simulink library "lib_affectiveChar_scenario"  (R2014a)
settings: Solver=ode45  StartTime=0.0  StopTime=10.0  RelTol=1e-3
values from neighbouring files (symbols this model uses):
  temp = sprintf('<face type=\"FACS\" side=\"BOTH\" au=\"    [cmdBML_AU.m]    (also in cmdBML_AU_VA.m; cmdBML_AUmerg.m; cmdBML_AUs.m)
undefined symbols (not defined in the file or in its folder): avert, bHand, boredom, BOREDOM_THRESHOLD, diff, GAZE_GUI, GAZE_SHOFTEYE, GAZE_USER_HAND, gazing, isPosing, p, r, randAvertGazeChance, randPoseChance, s, uHand
(part 1 of 2)
settings Model: Creator=Maryam  LastModifiedBy=root180

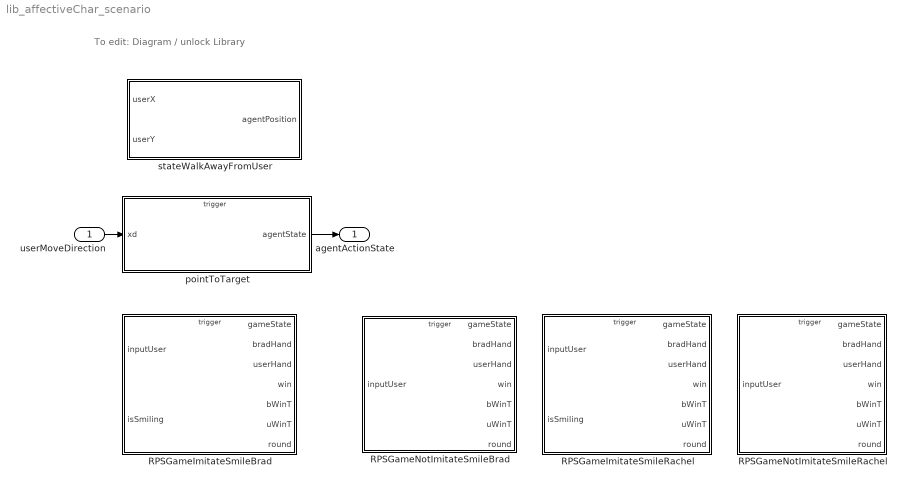
== system lib_affectiveChar_scenario ==
  note: To edit: Diagram / unlock Library
  userMoveDirection : Inport
  RPSGameImitateSmileBrad : Stateflow chart  TreatAsAtomicUnit=on
  RPSGameImitateSmileRachel : Stateflow chart  TreatAsAtomicUnit=on  DSMNames=BOREDOM_THRESHOLD,GAZE_GUI,GAZE_SHOFTEYE,GAZE_USER_HAND,avert,bHand,boredom,diff,gazing,isPosing,p,r,randAvertGazeChance,randPoseChance,s,temp,uHand  DSMValues=BOREDOM_THRESHOLD,GAZE_GUI,GAZE_SHOFTEYE,GAZE_USER_HAND,avert,bHand,boredom,diff,gazing,isPosing,p,r,randAvertGazeChance,randPoseChance,s,temp,uHand
  RPSGameNotImitateSmileBrad : Stateflow chart  TreatAsAtomicUnit=on
  RPSGameNotImitateSmileRachel : Stateflow chart  TreatAsAtomicUnit=on
  pointToTarget : Stateflow chart  TreatAsAtomicUnit=on
  stateWalkAwayFromUser : Stateflow chart  TreatAsAtomicUnit=on
  agentActionState : Outport
  wires:
  userMoveDirection/1 -> pointToTarget/1(xd)
  pointToTarget/1(agentState) -> agentActionState/1

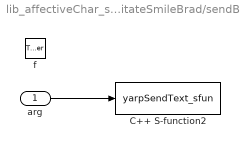
== system lib_affectiveChar_scenario/RPSGameImitateSmileBrad/sendBML ==
  arg : Inport  OutDataTypeStr=double  PortDimensions=[256 1]
  f : TriggerPort  TriggerType=function-call
      settings: CopyFcn=Stateflow.SLINSF.SimulinkMan.removeBlockPreDeleteFcn  PreDeleteFcn=Stateflow.SLINSF.SimulinkMan.unsafePredeleteFcn
  C++ S-function2 : S-Function  FunctionName=yarpSendText_sfun  Parameters='/sim/out/bml0', '/SB/in/bml'  EnableBusSupport=off
  wires:
  arg/1 -> C++ S-function2/1

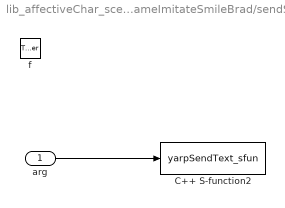
== system lib_affectiveChar_scenario/RPSGameImitateSmileBrad/sendSBM ==
  arg : Inport  OutDataTypeStr=double  PortDimensions=[256 1]
  f : TriggerPort  TriggerType=function-call
      settings: CopyFcn=Stateflow.SLINSF.SimulinkMan.removeBlockPreDeleteFcn  PreDeleteFcn=Stateflow.SLINSF.SimulinkMan.unsafePredeleteFcn
  C++ S-function2 : S-Function  FunctionName=yarpSendText_sfun  Parameters='/sim/out/smb0', '/SB/in/sbm'  EnableBusSupport=off
  wires:
  arg/1 -> C++ S-function2/1

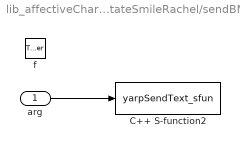
== system lib_affectiveChar_scenario/RPSGameImitateSmileRachel/sendBML ==
  arg : Inport  OutDataTypeStr=double  PortDimensions=[256 1]
  f : TriggerPort  TriggerType=function-call
      settings: CopyFcn=Stateflow.SLINSF.SimulinkMan.removeBlockPreDeleteFcn  PreDeleteFcn=Stateflow.SLINSF.SimulinkMan.unsafePredeleteFcn
  C++ S-function2 : S-Function  FunctionName=yarpSendText_sfun  Parameters='/sim/out/bml0', '/SB/in/bml'  EnableBusSupport=off
  wires:
  arg/1 -> C++ S-function2/1

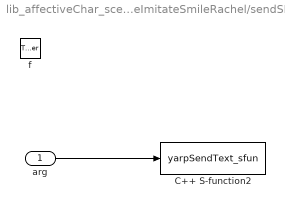
== system lib_affectiveChar_scenario/RPSGameImitateSmileRachel/sendSBM ==
  arg : Inport  OutDataTypeStr=double  PortDimensions=[256 1]
  f : TriggerPort  TriggerType=function-call
      settings: CopyFcn=Stateflow.SLINSF.SimulinkMan.removeBlockPreDeleteFcn  PreDeleteFcn=Stateflow.SLINSF.SimulinkMan.unsafePredeleteFcn
  C++ S-function2 : S-Function  FunctionName=yarpSendText_sfun  Parameters='/sim/out/smb0', '/SB/in/sbm'  EnableBusSupport=off
  wires:
  arg/1 -> C++ S-function2/1

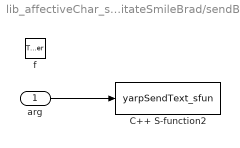
== system lib_affectiveChar_scenario/RPSGameNotImitateSmileBrad/sendBML ==
  arg : Inport  OutDataTypeStr=double  PortDimensions=[256 1]
  f : TriggerPort  TriggerType=function-call
      settings: CopyFcn=Stateflow.SLINSF.SimulinkMan.removeBlockPreDeleteFcn  PreDeleteFcn=Stateflow.SLINSF.SimulinkMan.unsafePredeleteFcn
  C++ S-function2 : S-Function  FunctionName=yarpSendText_sfun  Parameters='/sim/out/bml0', '/SB/in/bml'  EnableBusSupport=off
  wires:
  arg/1 -> C++ S-function2/1

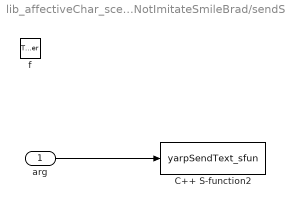
== system lib_affectiveChar_scenario/RPSGameNotImitateSmileBrad/sendSBM ==
  arg : Inport  OutDataTypeStr=double  PortDimensions=[256 1]
  f : TriggerPort  TriggerType=function-call
      settings: CopyFcn=Stateflow.SLINSF.SimulinkMan.removeBlockPreDeleteFcn  PreDeleteFcn=Stateflow.SLINSF.SimulinkMan.unsafePredeleteFcn
  C++ S-function2 : S-Function  FunctionName=yarpSendText_sfun  Parameters='/sim/out/smb0', '/SB/in/sbm'  EnableBusSupport=off
  wires:
  arg/1 -> C++ S-function2/1

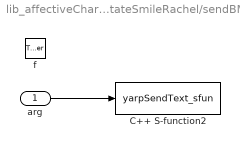
== system lib_affectiveChar_scenario/RPSGameNotImitateSmileRachel/sendBML ==
  arg : Inport  OutDataTypeStr=double  PortDimensions=[256 1]
  f : TriggerPort  TriggerType=function-call
      settings: CopyFcn=Stateflow.SLINSF.SimulinkMan.removeBlockPreDeleteFcn  PreDeleteFcn=Stateflow.SLINSF.SimulinkMan.unsafePredeleteFcn
  C++ S-function2 : S-Function  FunctionName=yarpSendText_sfun  Parameters='/sim/out/bml0', '/SB/in/bml'  EnableBusSupport=off
  wires:
  arg/1 -> C++ S-function2/1

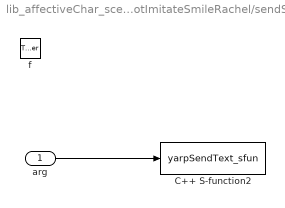
== system lib_affectiveChar_scenario/RPSGameNotImitateSmileRachel/sendSBM ==
  arg : Inport  OutDataTypeStr=double  PortDimensions=[256 1]
  f : TriggerPort  TriggerType=function-call
      settings: CopyFcn=Stateflow.SLINSF.SimulinkMan.removeBlockPreDeleteFcn  PreDeleteFcn=Stateflow.SLINSF.SimulinkMan.unsafePredeleteFcn
  C++ S-function2 : S-Function  FunctionName=yarpSendText_sfun  Parameters='/sim/out/smb0', '/SB/in/sbm'  EnableBusSupport=off
  wires:
  arg/1 -> C++ S-function2/1

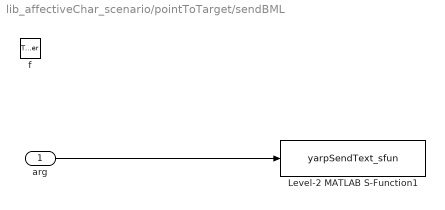
== system lib_affectiveChar_scenario/pointToTarget/sendBML ==
  arg : Inport  OutDataTypeStr=double  PortDimensions=[256 1]
  f : TriggerPort  TriggerType=function-call
      settings: CopyFcn=Stateflow.SLINSF.SimulinkMan.removeBlockPreDeleteFcn  PreDeleteFcn=Stateflow.SLINSF.SimulinkMan.unsafePredeleteFcn
  Level-2 MATLAB S-Function1 : M-S-Function  FunctionName=yarpSendText_sfun  Parameters='/sim/out/bml', '/SB/in/bml'
  wires:
  arg/1 -> Level-2 MATLAB S-Function1/1

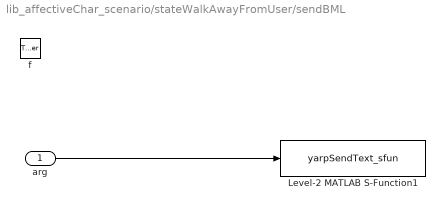
== system lib_affectiveChar_scenario/stateWalkAwayFromUser/sendBML ==
  arg : Inport  OutDataTypeStr=double  PortDimensions=[256 1]
  f : TriggerPort  TriggerType=function-call
      settings: CopyFcn=Stateflow.SLINSF.SimulinkMan.removeBlockPreDeleteFcn  PreDeleteFcn=Stateflow.SLINSF.SimulinkMan.unsafePredeleteFcn
  Level-2 MATLAB S-Function1 : M-S-Function  FunctionName=yarpSendText_sfun  Parameters='/sim/out/bml4', '/SB/in/bml'
  wires:
  arg/1 -> Level-2 MATLAB S-Function1/1

== stateflow chart lib_affectiveChar_scenario/stateWalkAwayFromUser ==
  state stateWalkAway
    entry:
    [arrBML,agentPosition ] = cmdBML_walkOppositeUser(userX, userY);
    sendBML(arrBML);
  state sendBML(arg) [function]
  data: arg function_input double size=[256 1]; userX input =5; userY input =5; agentPosition output double size=1; arrBML data_store_memory size=256

== stateflow chart lib_affectiveChar_scenario/RPSGameImitateSmileBrad ==
  state stateStart
    entry: round=0;avert=0;
    uHand=1; randSmile=0; userHand=3;bradHand=3; win=0;
    BOREDOM_THRESHOLD=10;
    gameState=0;randPoseChance=0;randAvertGazeChance=0;
    uWinT=0; bWinT=0; isPosing=0;
    boredom=0;
    sendBML(  initialPoseTable(1) );
  state sendSBM(arg) [function]
  state stateReady
    entry: round=round+1;
    bradHand=3;
    userHand=3;
    gameState= 0;
    win=0;isPosing=1;
  state sendBML(arg) [function]
  note: num of bmlID=2
  state gameOver
    entry: gameState=3;
    boredom=boredom-2;
  note: num of bmlID=2
  state statePoseReady
    entry:
    sendBML(  initialPoseTable(2) );
    sendSBM(handPoseSBTable(2));
    isPosing=1;
  note: num of bmlID=2
  state stateHeadNeutral2
    entry:
    sendBML( initialPoseTable(2 ) );
  note: num of sbmID=4
  note: num of bmlID=18
  state stateGo
    entry: isPosing=1;
    gameState= 1;
  state stateWinSmile
    entry:
    sendBML(successTable(1));
  note: num of bmlID=3
  state stateNeckBack
    entry: sendBML( successTable(2));
  state stateRandomHand
    entry: isPosing=1;
    bHand=randi([0,2]);
  state stateBrowUp
    entry:  sendBML( successTable(3));
  state statePoseFingersCLose
    entry:isPosing=1;
    sendSBM(handPoseSBTable(1));
  state stateNotWinBored
    entry:
    sendBML( idlePoseBradTable(randi([1,18])) );
  state statePosePaper
    entry: isPosing=1;p=randi([1,2]);
    sendBML(  paperPoseBradTable(p) );
  state statePoseRock
    entry: isPosing=1;r=randi([1,2]);
    sendBML(  rockPoseTable(r) );
  state statePoseScissors
    entry: isPosing=1; s=randi([1,2]);
    sendBML(  scissorsPoseBradTable(s) );
  state stateReadUserHand
    entry:isPosing=1;
    uHand=inputUser;
  state stateShowHands
    entry: isPosing=1;
    gameState=2;
    bradHand=bHand;
    userHand=uHand;
  state statePoseReturnFinger
    entry:isPosing=1;
    sendSBM(handPoseSBTable(2));
  state stateCompare
    entry:isPosing=1;
    temp=uHand-bHand;
    diff=temp- 3.*floor(temp/3);
  state stateUserWin
    entry:isPosing=0;
    win=1;
    uWinT=uWinT+1;
  state stateBradWin
    entry:isPosing=0;
    win=2;
    bWinT=bWinT+1;
  state stateNoWin
    entry:
    win=0;
    isPosing=0;
  state stateShowResult
    entry: isPosing=0;
  (default) -> stateStart
  stateStart -> stateReady : after(2,secs)
  stateReady -> stateReady [order 2] : [uHand==3]
  stateReady -> statePoseReady [order 1] : after(1,secs)[boredom<BOREDOM_THRESHOLD-4]{boredom=boredom+1;}
  (junction 2) -> stateReady [order 2] : after(3,secs)
  stateReady -> statePoseReady [order 3] : after(1,secs)
  (junction 2) -> gameOver [order 1] : after(3,secs)[round==10]
  stateShowResult -> (junction 2)
  gameOver -> stateHeadNeutral2
  stateHeadNeutral2 -> (junction 3) : after(1,secs)
  statePoseReady -> stateGo : after(3,secs)[uHand~=3]
  (junction 3) -> stateWinSmile [order 1] : [uWinT<bWinT]
  (junction 3) -> stateNotWinBored [order 2]
  stateWinSmile -> stateNeckBack : after(1,secs)
  stateGo -> stateRandomHand : after(1,secs)
  stateNeckBack -> stateBrowUp : after(1,secs)
  stateRandomHand -> (junction 5)
  (junction 5) -> statePoseFingersCLose [order 3] : [bHand==0]
  (junction 5) -> statePoseRock [order 2] : [bHand==2]
  (junction 5) -> statePosePaper [order 1] : [bHand==1]
  statePoseFingersCLose -> statePoseScissors
  statePoseRock -> stateReadUserHand : after(1,secs)[uHand~=3]
  statePosePaper -> stateReadUserHand : after(1,secs)[uHand~=3]
  statePoseScissors -> stateReadUserHand : after(1,secs)[uHand~=3]
  stateReadUserHand -> stateReadUserHand [order 1] : [uHand==3]
  stateReadUserHand -> statePoseReturnFinger [order 2] : [bHand==0]
  stateReadUserHand -> stateShowHands [order 3]
  statePoseReturnFinger -> stateShowHands
  stateShowHands -> stateCompare
  stateCompare -> stateUserWin [order 2] : [diff==2]
  stateCompare -> stateBradWin [order 1] : [diff==1]
  stateCompare -> stateNoWin [order 3] : [diff~=1 && diff~=2]
  stateBradWin -> stateShowResult
  stateNoWin -> stateShowResult : after(5,secs)
  stateUserWin -> stateShowResult : after(5,secs)
  data: arg function_input double size=[256 1]; arg function_input double size=[256 1]; bmlID function_input double; poseBML function_output double size=[256,1]; bmlID function_input double; poseBML function_output double size=[256,1]; bmlID function_input double; poseBML function_output double size=[256,1]; sbmID function_input double; poseSBM function_output double size=[256,1]; bmlID function_input double; poseBML function_output double size=[256,1]; bmlID function_input double; poseBML function_output double size=[256,1]; bmlID function_input double; poseBML function_output double size=[256,1]; gameState output double size=1 =0; inputUser input double size=1; bradHand output double size=1; userHand output double size=1 =3; win output double size=1; temp data_store_memory size=2; diff data_store_memory size=2; uHand data_store_memory size=2; bHand data_store_memory size=2; bWinT output double size=1; uWinT output double size=1; smileN data_store_memory size=2; randSmile data_store_memory size=2; boredom data_store_memory size=2; BOREDOM_THRESHOLD data_store_memory size=2; randAvertGazeChance data_store_memory size=2; randPoseChance data_store_memory size=2; isPosing data_store_memory size=2; r data_store_memory size=2; p data_store_memory size=2; s data_store_memory size=2; round output double size=1 =0; isSmiling input double size=1; avert data_store_memory
  events: secs input RISING_EDGE_EVENT
  function poseBML = rockPoseTable(bmlID):
    | function poseBML = rockPoseTable(bmlID)
    | 
    | aVarTruthTableCondition_1 = false;
    | aVarTruthTableCondition_2 = false;
    | 
    | 
    | % rock
    | 
    | aVarTruthTableCondition_1 = logical(bmlID==1);
    | 
    | % rock
    | 
    | aVarTruthTableCondition_2 = logical(bmlID==2);
    | 
    | if (aVarTruthTableCondition_1)
    |     aFcnTruthTableAction_1();
    | elseif (aVarTruthTableCondition_2)
    |     aFcnTruthTableAction_2();
    | else % Default
    |     aFcnTruthTableAction_1();
    | end
    | 
    | function aFcnTruthTableAction_1()
    | 
    | % rock
    | 
    | poseBML=encStr2Arr('<?xml version="1.0" ?><act><bml><animation name="ChrBrad@Idle01_BeatFistMidLf02"/></bml></act>');
    | 
    | function aFcnTruthTableAction_2()
    | 
    | % rock2
    | 
    | poseBML=encStr2Arr('<?xml version="1.0" ?><act><bml><animation name="ChrBrad@Idle01_BeatFistMidLf01"/></bml></act>');
  function poseBML = paperPoseBradTable(bmlID):
    | function poseBML = paperPoseBradTable(bmlID)
    | 
    | aVarTruthTableCondition_1 = false;
    | aVarTruthTableCondition_2 = false;
    | 
    | 
    | % paper
    | 
    | aVarTruthTableCondition_1 = logical(bmlID==1);
    | 
    | % paper2
    | 
    | aVarTruthTableCondition_2 = logical(bmlID==2);
    | 
    | if (aVarTruthTableCondition_1)
    |     aFcnTruthTableAction_1();
    | elseif (aVarTruthTableCondition_2)
    |     aFcnTruthTableAction_2();
    | else % Default
    |     aFcnTruthTableAction_2();
    | end
    | 
    | function aFcnTruthTableAction_1()
    | 
    | % paper
    | 
    | poseBML=encStr2Arr('<?xml version="1.0" ?><act><bml><animation name="ChrBrad@Idle01_OfferLf01"/></bml></act>');
    | 
    | function aFcnTruthTableAction_2()
    | 
    | % paper2
    | 
    | poseBML=encStr2Arr('<?xml version="1.0" ?><act><bml><animation name="ChrBrad@Idle01_YouLf01"/></bml></act>');
  function poseBML = scissorsPoseBradTable(bmlID):
    | function poseBML = scissorsPoseBradTable(bmlID)
    | 
    | aVarTruthTableCondition_1 = false;
    | aVarTruthTableCondition_2 = false;
    | 
    | 
    | % scissors
    | 
    | aVarTruthTableCondition_1 = logical(bmlID==1);
    | 
    | % scissors2
    | 
    | aVarTruthTableCondition_2 = logical(bmlID==2);
    | 
    | if (aVarTruthTableCondition_1)
    |     aFcnTruthTableAction_1();
    | elseif (aVarTruthTableCondition_2)
    |     aFcnTruthTableAction_2();
    | else % Default
    |     aFcnTruthTableAction_1();
    | end
    | 
    | function aFcnTruthTableAction_1()
    | 
    | % scissors
    | 
    | poseBML=encStr2Arr('<?xml version="1.0" ?><act><bml><animation name="ChrBrad@Idle01_YouLf01"/></bml></act>');
    | 
    | function aFcnTruthTableAction_2()
    | 
    | % scissors2
    | 
    | poseBML=encStr2Arr('<?xml version="1.0" ?><act><bml><animation name="ChrBrad@Idle01_OfferLf01"/></bml></act>');
  function poseSBM = handPoseSBTable(sbmID):
    | function poseSBM = handPoseSBTable(sbmID)
    | 
    | aVarTruthTableCondition_1 = false;
    | aVarTruthTableCondition_2 = false;
    | aVarTruthTableCondition_3 = false;
    | aVarTruthTableCondition_4 = false;
    | 
    | 
    | % fingersClose
    | 
    | aVarTruthTableCondition_1 = logical(sbmID==1);
    | 
    | % fingersNeutral
    | 
    | aVarTruthTableCondition_2 = logical(sbmID==2);
    | 
    | % lshoulkderForward
    | 
    | aVarTruthTableCondition_3 = logical(sbmID==3);
    | 
    | % lshoulkderNeutral
    | 
    | aVarTruthTableCondition_4 = logical(sbmID==4);
    | 
    | if (aVarTruthTableCondition_1)
    |     aFcnTruthTableAction_1();
    | elseif (aVarTruthTableCondition_2)
    |     aFcnTruthTableAction_2();
    | elseif (aVarTruthTableCondition_3)
    |     aFcnTruthTableAction_3();
    | elseif (aVarTruthTableCondition_4)
    |     aFcnTruthTableAction_4();
    | else % Default
    |     aFcnTruthTableAction_1();
    | end
    | 
    | function aFcnTruthTableAction_1()
    | 
    | % fingersClose
    | 
    | poseSBM=encStr2Arr('brad.getSkeleton().getJointByName("l_pinky1").setPostrotation(SrQuat(1,0,0,0.5)); brad.getSkeleton().getJointByName("l_ring1").setPostrotation(SrQuat(1,0,0,0.5))');
    | 
    | function aFcnTruthTableAction_2()
    | 
    | % fingersNeutral
    | 
    | poseSBM=encStr2Arr('brad.getSkeleton().getJointByName("l_pinky1").setPostrotation(SrQuat(1,0,0,0)); brad.getSkeleton().getJointByName("l_ring1").setPostrotation(SrQuat(1,0,0,0))');
    | 
    | function aFcnTruthTableAction_3()
    | 
    | % lshoulkderForward
    | 
    | poseSBM=encStr2Arr('brad.getSkeleton().getJointByName("l_sternoclavicular").setPostrotation(SrQuat(1,0,0,0.05))');
    | 
    | function aFcnTruthTableAction_4()
    | 
    | % lshoulkderNeutral
    | 
    | poseSBM=encStr2Arr('brad.getSkeleton().getJointByName("l_sternoclavicular").setPostrotation(SrQuat(1,0,0,0))');
  function poseBML=idlePoseBradTable(bmlID):
    | function poseBML=idlePoseBradTable(bmlID)
    | 
    | aVarTruthTableCondition_1 = false;
    | aVarTruthTableCondition_2 = false;
    | aVarTruthTableCondition_3 = false;
    | aVarTruthTableCondition_4 = false;
    | aVarTruthTableCondition_5 = false;
    | aVarTruthTableCondition_6 = false;
    | aVarTruthTableCondition_7 = false;
    | aVarTruthTableCondition_8 = false;
    | aVarTruthTableCondition_9 = false;
    | aVarTruthTableCondition_10 = false;
    | aVarTruthTableCondition_11 = false;
    | aVarTruthTableCondition_12 = false;
    | aVarTruthTableCondition_13 = false;
    | aVarTruthTableCondition_14 = false;
    | aVarTruthTableCondition_15 = false;
    | aVarTruthTableCondition_16 = false;
    | aVarTruthTableCondition_17 = false;
    | aVarTruthTableCondition_18 = false;
    | 
    | 
    | 
    | aVarTruthTableCondition_1 = logical(bmlID==1);
    | 
    | 
    | aVarTruthTableCondition_2 = logical(bmlID==2);
    | 
    | 
    | aVarTruthTableCondition_3 = logical(bmlID==3);
    | 
    | 
    | aVarTruthTableCondition_4 = logical(bmlID==4);
    | 
    | 
    | aVarTruthTableCondition_5 = logical(bmlID==5);
    | 
    | 
    | aVarTruthTableCondition_6 = logical(bmlID==6);
    | 
    | 
    | aVarTruthTableCondition_7 = logical(bmlID==7);
    | 
    | 
    | aVarTruthTableCondition_8 = logical(bmlID==8);
    | 
    | 
    | aVarTruthTableCondition_9 = logical(bmlID==9);
    | 
    | 
    | aVarTruthTableCondition_10 = logical(bmlID==10);
    | 
    | 
    | aVarTruthTableCondition_11 = logical(bmlID==11);
    | 
    | 
    | aVarTruthTableCondition_12 = logical(bmlID==12);
    | 
    | 
    | aVarTruthTableCondition_13 = logical(bmlID==13);
    | 
    | 
    | aVarTruthTableCondition_14 = logical(bmlID==14);
    | 
    | 
    | aVarTruthTableCondition_15 = logical(bmlID==15);
    | 
    | 
    | aVarTruthTableCondition_16 = logical(bmlID==16);
    | 
    | 
    | aVarTruthTableCondition_17 = logical(bmlID==17);
    | 
    | 
    | aVarTruthTableCondition_18 = logical(bmlID==18);
    | 
    | if (aVarTruthTableCondition_1)
    |     aFcnTruthTableAction_1();
    | elseif (aVarTruthTableCondition_2)
    |     aFcnTruthTableAction_2();
    | elseif (aVarTruthTableCondition_3)
    |     aFcnTruthTableAction_3();
    | elseif (aVarTruthTableCondition_4)
    |     aFcnTruthTableAction_4();
    | elseif (aVarTruthTableCondition_5)
    |     aFcnTruthTableAction_5();
    | elseif (aVarTruthTableCondition_6)
    |     aFcnTruthTableAction_11();
    | elseif (aVarTruthTableCondition_7)
    |     aFcnTruthTableAction_3();
    | elseif (aVarTruthTableCondition_8)
    |     aFcnTruthTableAction_5();
    | elseif (aVarTruthTableCondition_9)
    |     aFcnTruthTableAction_3();
    | elseif (aVarTruthTableCondition_10)
    |     aFcnTruthTableAction_10();
    | elseif (aVarTruthTableCondition_11)
    |     aFcnTruthTableAction_11();
    | elseif (aVarTruthTableCondition_12)
    |     aFcnTruthTableAction_8();
    | elseif (aVarTruthTableCondition_13)
    |     aFcnTruthTableAction_8();
    | elseif (aVarTruthTableCondition_14)
    |     aFcnTruthTableAction_7();
    | elseif (aVarTruthTableCondition_15)
    |     aFcnTruthTableAction_6();
    | elseif (aVarTruthTableCondition_16)
    |     aFcnTruthTableAction_5();
    | elseif (aVarTruthTableCondition_17)
    |     aFcnTruthTableAction_8();
    | elseif (aVarTruthTableCondition_18)
    |     aFcnTruthTableAction_9();
    | else % Default
    |     aFcnTruthTableAction_3();
    | end
    | 
    | function aFcnTruthTableAction_1()
    | 
    | % ArmStretchHandsFW
    | 
    | poseBML=encStr2Arr('<?xml version="1.0" ?><act><bml><animation name="ChrBrad@Idle01_ArmStretch01"/></bml></act>');
    | 
    | function aFcnTruthTableAction_2()
    | 
    | % HandsOnWaist
    | 
    | poseBML=encStr2Arr('<?xml version="1.0" ?><act><bml><animation name="ChrBrad@Idle01_ToIdle03"/></bml></act>');
    | 
    | function aFcnTruthTableAction_3()
    | 
    | % WeightShift
    | 
    | poseBML=encStr2Arr('<?xml version="1.0" ?><act><bml><animation name="ChrBrad@Idle01_WeightShift01" /></bml></act>');
    | 
    | function aFcnTruthTableAction_4()
    | 
    | % ScratchChest
    | 
    | poseBML=encStr2Arr('<?xml version="1.0" ?><act><bml><animation name="ChrBrad@Idle01_ScratchChest01" /></bml></act>');
    | 
    | function aFcnTruthTableAction_5()
    | 
    | % ScratchHead
    | 
    | poseBML=encStr2Arr('<?xml version="1.0" ?><act><bml><animation name="ChrBrad@Idle01_ScratchHeadLf01" /></bml></act>');
    | 
    | function aFcnTruthTableAction_6()
    | 
    | % ShoulderStretchUpDown
    | 
    | poseBML=encStr2Arr('<?xml version="1.0" ?><act><bml><animation name="ChrBrad@Idle01_ShoulderStretch01" /></bml></act>');
    | 
    | function aFcnTruthTableAction_7()
    | 
    | % scratchtemple(head)
    | 
    | poseBML=encStr2Arr('<?xml version="1.0" ?><act><bml><animation name="ChrBrad@Idle01_ScratchTempleLf01" /></bml></act>');
    | 
    | function aFcnTruthTableAction_8()
    | 
    | % SqueezeHand01
    | 
    | poseBML=encStr2Arr('<?xml version="1.0" ?><act><bml><animation name="ChrBrad@Idle01_SqueezeHand01" /></bml></act>');
    | 
    | function aFcnTruthTableAction_9()
    | 
    | % TouchHands01
    | 
    | poseBML=encStr2Arr('<?xml version="1.0" ?><act><bml><animation name="ChrBrad@Idle01_TouchHands01" /></bml></act>');
    | 
    | function aFcnTruthTableAction_10()
    | 
    | % WeightShift2
    | 
    | poseBML=encStr2Arr('<?xml version="1.0" ?><act><bml><animation name="ChrBrad@Idle01_WeightShift02" /></bml></act>');
    | 
    | function aFcnTruthTableAction_11()
    | 
    | % Idle01_ToIdle02
    | 
    | poseBML=encStr2Arr('<?xml version="1.0" ?><act><bml><animation name="ChrBrad@Idle01_ToIdle02" /></bml></act>');
  function poseBML=initialPoseTable(bmlID):
    | function poseBML=initialPoseTable(bmlID)
    | 
    | aVarTruthTableCondition_1 = false;
    | aVarTruthTableCondition_2 = false;
    | aVarTruthTableCondition_3 = false;
    | 
    | 
    | 
    | aVarTruthTableCondition_1 = logical(bmlID==1);
    | 
    | 
    | aVarTruthTableCondition_2 = logical(bmlID==2);
    | 
    | 
    | aVarTruthTableCondition_3 = logical(bmlID==3);
    | 
    | if (aVarTruthTableCondition_1)
    |     aFcnTruthTableAction_1();
    | elseif (aVarTruthTableCondition_2)
    |     aFcnTruthTableAction_2();
    | elseif (aVarTruthTableCondition_3)
    |     aFcnTruthTableAction_3();
    | else % Default
    |     aFcnTruthTableAction_1();
    | end
    | 
    | function aFcnTruthTableAction_1()
    | 
    | % saccadeFinish
    | 
    | poseBML=encStr2Arr('<?xml version="1.0" ?><act><bml><saccade finish="true"/></bml></act>');
    | 
    | function aFcnTruthTableAction_2()
    | 
    | % neutralHeadGaze
    | 
    | poseBML=encStr2Arr('<?xml version="1.0" ?><act><bml><gaze target="camera" sbm:time-hint="0.2"/></bml></act>');
    | 
    | function aFcnTruthTableAction_3()
    | 
    | % blink
    | 
    | poseBML=encStr2Arr('<?xml version="1.0" ?><act><bml><face type="FACS" side="BOTH" au="45" amount="0.5" /></bml></act>');
  function poseBML = successTable(bmlID):
    | function poseBML = successTable(bmlID)
    | 
    | aVarTruthTableCondition_1 = false;
    | aVarTruthTableCondition_2 = false;
    | aVarTruthTableCondition_3 = false;
    | 
    | 
    | % smile
    | 
    | aVarTruthTableCondition_1 = logical(bmlID==1);
    | 
    | % HeadChestUp
    | 
    | aVarTruthTableCondition_2 = logical(bmlID==2);
    | 
    | % browUp
    | 
    | aVarTruthTableCondition_3 = logical(bmlID==3);
    | 
    | if (aVarTruthTableCondition_1)
    |     aFcnTruthTableAction_1();
    | elseif (aVarTruthTableCondition_2)
    |     aFcnTruthTableAction_2();
    | elseif (aVarTruthTableCondition_3)
    |     aFcnTruthTableAction_3();
    | else % Default
    |     aFcnTruthTableAction_1();
    | end
    | 
    | function aFcnTruthTableAction_1()
    | 
    | % smile
    | 
    | poseBML=encStr2Arr('<?xml version="1.0" ?><act><bml><face amount="1" au="12" end="8" relax="6" side="BOTH" start="0" stroke="3" type="facs"/><face amount="0.5" au="6" end="8" relax="6" side="BOTH" start="0" stroke="3" type="facs"/></bml></act>');
    | 
    | function aFcnTruthTableAction_2()
    | 
    | % HeadChestUp
    | 
    | poseBML=encStr2Arr('<?xml version="1.0" ?><act><bml><gaze angle="12" direction="UP" sbm:joint-range="HEAD CHEST" sbm:time-hint="0.3" target="camera"/></bml></act>');
    | 
    | function aFcnTruthTableAction_3()
    | 
    | % browUp
    | 
    | poseBML=encStr2Arr('<?xml version="1.0" ?><act><bml><face amount="0.3" au="1" end="6" side="BOTH" start="0" type="facs"/><face amount="0.8"  au="2" end="6" side="BOTH" start="0" type="facs"/></bml></act>');

== stateflow chart lib_affectiveChar_scenario/RPSGameNotImitateSmileRachel ==
  state stateStart
    entry:
    BOREDOM_THRESHOLD=10;
    round=0;avert=0;uHand=1; bHand=1; bradHand=3; userHand=3;
    win=0; gameState=0;uWinT=0; bWinT=0; isPosing=0; isSmiling=0; randSmile=0;
    boredom=0;randAvertGazeChance=0;randPoseChance=0;
    sendBML(  initialPoseTable(1) );
  state sendSBM(arg) [function]
  state sendBML(arg) [function]
  state stateReady
    entry: round=round+1;
    bradHand=3;
    userHand=3;
    gameState= 0;
    win=0;isPosing=1;
  state gameOver
    entry: gameState=3;
    boredom=boredom-2;
  note: num of bmlID=2
  state statePoseReady
    entry:
    sendBML(  initialPoseTable(2) );
    sendSBM(handPoseSBRachelTable(2));
    isPosing=1;
  state stateHeadNeutral2
    entry:
    sendBML(  initialPoseTable(2) );
  state stateIfSmile
    entry: randSmile=randi([0,boredom]);
    isPosing=1;
  note: num of bmlID=18
  state stateGo
    entry: isPosing=1;
    gameState= 1;
    isSmiling=0;
  state stateSmile
    entry: isSmiling=1;
  state statePoseSmile
    entry: isSmiling=1;
  note: num of bmlID=3
  state stateNeckBack
    entry: sendBML( successTable(2));
    isSmiling=0;
  state stateRandomHand
    entry: isPosing=1;
    bHand=randi([0,2]);
  state stateBrowUp
    entry:  sendBML( successTable(3));
  state stateBoredPose1
    entry:
    sendBML( idlePoseRachelTable(randi([1,18])) );
  state statePoseFingersCLose
    entry:isPosing=1;
    sendSBM(handPoseSBRachelTable(1));
  state statePosePaper
    entry: isPosing=1;
    sendBML(  paperPoseRachelTable(1) );
  state statePoseRock
    entry: isPosing=1;r=randi([1,2]);
    sendBML(  rockPoseTable(r) );
  state statePoseScissors
    entry: isPosing=1;
    sendBML(  scissorsPoseRachelTable(1) );
  state stateReadUserHand
    entry:isPosing=1;
    uHand=inputUser;
  state stateShowHands
    entry: isPosing=1;
    gameState=2;
    bradHand=bHand;
    userHand=uHand;
  state statePoseReturnFinger
    entry:isPosing=1;
    sendSBM(handPoseSBRachelTable(2));
  state stateCompare
    entry:isPosing=1;
    temp=uHand-bHand;
    diff=temp- 3.*floor(temp/3);
  state stateUserWin
    entry:isPosing=0;
    win=1;
    uWinT=uWinT+1;
  state stateBradWin
    entry:isPosing=0;
    win=2;
    bWinT=bWinT+1;
  state stateNoWin
    entry:
    win=0;
    isPosing=0;
  state stateRandom1
    entry: randSmile=randi([0,boredom]);
    isPosing=0;
  state stateHeadNeutral1
    entry:
    sendBML(  initialPoseTable(2) );
  state statePoseSmileWin
    entry:isSmiling=1;
    isPosing=1;
  state stateShowResult
    entry: isPosing=0;
    isSmiling=0;
  (default) -> stateStart
  stateStart -> stateReady : after(2,secs)
  stateReady -> stateReady [order 2] : [uHand==3]
  stateReady -> statePoseReady [order 1] : after(1,secs)[boredom<BOREDOM_THRESHOLD-4]{boredom=boredom+1;}
  (junction 2) -> gameOver [order 1] : after(3,secs)[round==10]
  (junction 2) -> stateReady [order 2] : after(3,secs)
  stateShowResult -> (junction 2)
  stateReady -> statePoseReady [order 3] : after(1,secs)
  gameOver -> stateHeadNeutral2
  statePoseReady -> stateIfSmile : after(3,secs)[uHand~=3]
  stateHeadNeutral2 -> (junction 3) : after(1,secs)
  stateIfSmile -> (junction 4) [order 2] : [randSmile~=1]
  (junction 3) -> stateBoredPose1 [order 2]
  stateIfSmile -> statePoseSmile [order 1] : [randSmile==1]
  (junction 3) -> stateSmile [order 1] : [uWinT<bWinT]
  (junction 4) -> stateGo
  statePoseSmile -> (junction 4)
  stateGo -> stateRandomHand : after(1,secs)
  stateSmile -> stateNeckBack : after(1,secs)
  stateNeckBack -> stateBrowUp : after(1,secs)
  stateRandomHand -> (junction 5)
  (junction 5) -> statePoseRock [order 2] : [bHand==2]
  (junction 5) -> statePosePaper [order 1] : [bHand==1]
  (junction 5) -> statePoseFingersCLose [order 3] : [bHand==0]
  statePoseFingersCLose -> statePoseScissors
  statePoseRock -> stateReadUserHand : after(1,secs)[uHand~=3]
  statePosePaper -> stateReadUserHand : after(1,secs)[uHand~=3]
  statePoseScissors -> stateReadUserHand : after(1,secs)[uHand~=3]
  stateReadUserHand -> stateReadUserHand [order 1] : [uHand==3]
  stateReadUserHand -> stateShowHands [order 3]
  stateReadUserHand -> statePoseReturnFinger [order 2] : [bHand==0]
  statePoseReturnFinger -> stateShowHands
  stateShowHands -> stateCompare
  stateCompare -> stateUserWin [order 2] : [diff==2]
  stateCompare -> stateBradWin [order 1] : [diff==1]
  stateCompare -> stateNoWin [order 3] : [diff~=1 && diff~=2]
  stateBradWin -> stateRandom1
  stateNoWin -> stateRandom1 : after(5,secs)
  stateUserWin -> stateRandom1 : after(5,secs)
  stateRandom1 -> stateHeadNeutral1 [order 1] : [randSmile==1]
  stateRandom1 -> stateShowResult [order 2] : [randSmile~=1]
  stateHeadNeutral1 -> statePoseSmileWin : after(1,secs)
  statePoseSmileWin -> stateShowResult : after(5,secs)
  data: arg function_input double size=[256 1]; arg function_input double size=[256 1]; bmlID function_input double; poseBML function_output double size=[256,1]; bmlID function_input double; poseBML function_output double size=[256,1]; bmlID function_input double; poseBML function_output double size=[256,1]; sbmID function_input double; poseSBM function_output double size=[256,1]; bmlID function_input double; poseBML function_output double size=[256,1]; bmlID function_input double; poseBML function_output double size=[256,1]; bmlID function_input double; poseBML function_output double size=[256,1]; gameState output double size=1 =0; inputUser input double size=1; bradHand output double size=1; userHand output double size=1 =3; win output double size=1; temp data_store_memory size=2; diff data_store_memory size=2; uHand data_store_memory size=2; bHand data_store_memory size=2; bWinT output double size=1; uWinT output double size=1; randSmile data_store_memory size=2; boredom data_store_memory size=2; BOREDOM_THRESHOLD data_store_memory size=2; randAvertGazeChance data_store_memory size=2; randPoseChance data_store_memory size=2; isPosing data_store_memory size=2; r data_store_memory size=2; p data_store_memory size=2; s data_store_memory size=2; wristRotate data_store_memory size=2; round output double size=1 =0; isSmiling data_store_memory; avert data_store_memory
  events: secs input RISING_EDGE_EVENT
  function poseBML = paperPoseRachelTable(bmlID):
    | function poseBML = paperPoseRachelTable(bmlID)
    | 
    | aVarTruthTableCondition_1 = false;
    | 
    | 
    | % paper
    | 
    | aVarTruthTableCondition_1 = logical(bmlID==1);
    | 
    | if (aVarTruthTableCondition_1)
    |     aFcnTruthTableAction_1();
    | else % Default
    |     aFcnTruthTableAction_1();
    | end
    | 
    | function aFcnTruthTableAction_1()
    | 
    | % paper
    | 
    | poseBML=encStr2Arr('<?xml version="1.0" ?><act><bml><animation name="ChrBrad@Idle01_YouLf01"/></bml></act>');
  function poseBML = scissorsPoseRachelTable(bmlID):
    | function poseBML = scissorsPoseRachelTable(bmlID)
    | 
    | aVarTruthTableCondition_1 = false;
    | 
    | 
    | % scissors
    | 
    | aVarTruthTableCondition_1 = logical(bmlID==1);
    | 
    | if (aVarTruthTableCondition_1)
    |     aFcnTruthTableAction_1();
    | else % Default
    |     aFcnTruthTableAction_1();
    | end
    | 
    | function aFcnTruthTableAction_1()
    | 
    | % scissors
    | 
    | poseBML=encStr2Arr('<?xml version="1.0" ?><act><bml><animation name="ChrBrad@Idle01_YouLf01"/></bml></act>');
  function poseBML = rockPoseTable(bmlID):
    | function poseBML = rockPoseTable(bmlID)
    | 
    | aVarTruthTableCondition_1 = false;
    | aVarTruthTableCondition_2 = false;
    | 
    | 
    | % rock
    | 
    | aVarTruthTableCondition_1 = logical(bmlID==1);
    | 
    | % rock
    | 
    | aVarTruthTableCondition_2 = logical(bmlID==2);
    | 
    | if (aVarTruthTableCondition_1)
    |     aFcnTruthTableAction_1();
    | elseif (aVarTruthTableCondition_2)
    |     aFcnTruthTableAction_2();
    | else % Default
    |     aFcnTruthTableAction_1();
    | end
    | 
    | function aFcnTruthTableAction_1()
    | 
    | % rock
    | 
    | poseBML=encStr2Arr('<?xml version="1.0" ?><act><bml><animation name="ChrBrad@Idle01_BeatFistMidLf02"/></bml></act>');
    | 
    | function aFcnTruthTableAction_2()
    | 
    | % rock2
    | 
    | poseBML=encStr2Arr('<?xml version="1.0" ?><act><bml><animation name="ChrBrad@Idle01_BeatFistMidLf01"/></bml></act>');
  function poseSBM = handPoseSBRachelTable(sbmID):
    | function poseSBM = handPoseSBRachelTable(sbmID)
    | 
    | aVarTruthTableCondition_1 = false;
    | aVarTruthTableCondition_2 = false;
    | aVarTruthTableCondition_3 = false;
    | aVarTruthTableCondition_4 = false;
    | 
    | 
    | % fingersClose
    | 
    | aVarTruthTableCondition_1 = logical(sbmID==1);
    | 
    | % fingersNeutral
    | 
    | aVarTruthTableCondition_2 = logical(sbmID==2);
    | 
    | % lshoulkderForward
    | 
    | aVarTruthTableCondition_3 = logical(sbmID==3);
    | 
    | % lshoulkderNeutral
    | 
    | aVarTruthTableCondition_4 = logical(sbmID==4);
    | 
    | if (aVarTruthTableCondition_1)
    |     aFcnTruthTableAction_1();
    | elseif (aVarTruthTableCondition_2)
    |     aFcnTruthTableAction_2();
    | elseif (aVarTruthTableCondition_3)
    |     aFcnTruthTableAction_3();
    | elseif (aVarTruthTableCondition_4)
    |     aFcnTruthTableAction_4();
    | else % Default
    |     aFcnTruthTableAction_1();
    | end
    | 
    | function aFcnTruthTableAction_1()
    | 
    | % fingersClose
    | 
    | poseSBM=encStr2Arr('Rachel.getSkeleton().getJointByName("l_pinky1").setPostrotation(SrQuat(1,0,0,0.5)); Rachel.getSkeleton().getJointByName("l_ring1").setPostrotation(SrQuat(1,0,0,0.5))');
    | 
    | function aFcnTruthTableAction_2()
    | 
    | % fingersNeutral
    | 
    | poseSBM=encStr2Arr('Rachel.getSkeleton().getJointByName("l_pinky1").setPostrotation(SrQuat(1,0,0,0)); Rachel.getSkeleton().getJointByName("l_ring1").setPostrotation(SrQuat(1,0,0,0))');
    | 
    | function aFcnTruthTableAction_3()
    | 
    | % lshoulkderForward
    | 
    | poseSBM=encStr2Arr('Rachel.getSkeleton().getJointByName("l_sternoclavicular").setPostrotation(SrQuat(1,0,0,0.05))');
    | 
    | function aFcnTruthTableAction_4()
    | 
    | % lshoulkderNeutral
    | 
    | poseSBM=encStr2Arr('Rachel.getSkeleton().getJointByName("l_sternoclavicular").setPostrotation(SrQuat(1,0,0,0))');
  function poseBML=idlePoseRachelTable(bmlID):
    | function poseBML=idlePoseRachelTable(bmlID)
    | 
    | aVarTruthTableCondition_1 = false;
    | aVarTruthTableCondition_2 = false;
    | aVarTruthTableCondition_3 = false;
    | aVarTruthTableCondition_4 = false;
    | aVarTruthTableCondition_5 = false;
    | aVarTruthTableCondition_6 = false;
    | aVarTruthTableCondition_7 = false;
    | aVarTruthTableCondition_8 = false;
    | aVarTruthTableCondition_9 = false;
    | aVarTruthTableCondition_10 = false;
    | aVarTruthTableCondition_11 = false;
    | aVarTruthTableCondition_12 = false;
    | aVarTruthTableCondition_13 = false;
    | aVarTruthTableCondition_14 = false;
    | aVarTruthTableCondition_15 = false;
    | aVarTruthTableCondition_16 = false;
    | aVarTruthTableCondition_17 = false;
    | aVarTruthTableCondition_18 = false;
    | 
    | 
    | 
    | aVarTruthTableCondition_1 = logical(bmlID==1);
    | 
    | 
    | aVarTruthTableCondition_2 = logical(bmlID==2);
    | 
    | 
    | aVarTruthTableCondition_3 = logical(bmlID==3);
    | 
    | 
    | aVarTruthTableCondition_4 = logical(bmlID==4);
    | 
    | 
    | aVarTruthTableCondition_5 = logical(bmlID==5);
    | 
    | 
    | aVarTruthTableCondition_6 = logical(bmlID==6);
    | 
    | 
    | aVarTruthTableCondition_7 = logical(bmlID==7);
    | 
    | 
    | aVarTruthTableCondition_8 = logical(bmlID==8);
    | 
    | 
    | aVarTruthTableCondition_9 = logical(bmlID==9);
    | 
    | 
    | aVarTruthTableCondition_10 = logical(bmlID==10);
    | 
    | 
    | aVarTruthTableCondition_11 = logical(bmlID==11);
    | 
    | 
    | aVarTruthTableCondition_12 = logical(bmlID==12);
    | 
    | 
    | aVarTruthTableCondition_13 = logical(bmlID==13);
    | 
    | 
    | aVarTruthTableCondition_14 = logical(bmlID==14);
    | 
    | 
    | aVarTruthTableCondition_15 = logical(bmlID==15);
    | 
    | 
    | aVarTruthTableCondition_16 = logical(bmlID==16);
    | 
    | 
    | aVarTruthTableCondition_17 = logical(bmlID==17);
    | 
    | 
    | aVarTruthTableCondition_18 = logical(bmlID==18);
    | 
    | if (aVarTruthTableCondition_1)
    |     aFcnTruthTableAction_7();
    | elseif (aVarTruthTableCondition_2)
    |     aFcnTruthTableAction_2();
    | elseif (aVarTruthTableCondition_3)
    |     aFcnTruthTableAction_1();
    | elseif (aVarTruthTableCondition_4)
    |     aFcnTruthTableAction_2();
    | elseif (aVarTruthTableCondition_5)
    |     aFcnTruthTableAction_3();
    | elseif (aVarTruthTableCondition_6)
    |     aFcnTruthTableAction_8();
    | elseif (aVarTruthTableCondition_7)
    |     aFcnTruthTableAction_1();
    | elseif (aVarTruthTableCondition_8)
    |     aFcnTruthTableAction_3();
    | elseif (aVarTruthTableCondition_9)
    |     aFcnTruthTableAction_1();
    | elseif (aVarTruthTableCondition_10)
    |     aFcnTruthTableAction_7();
    | elseif (aVarTruthTableCondition_11)
    |     aFcnTruthTableAction_8();
    | elseif (aVarTruthTableCondition_12)
    |     aFcnTruthTableAction_6();
    | elseif (aVarTruthTableCondition_13)
    |     aFcnTruthTableAction_6();
    | elseif (aVarTruthTableCondition_14)
    |     aFcnTruthTableAction_5();
    | elseif (aVarTruthTableCondition_15)
    |     aFcnTruthTableAction_4();
    | elseif (aVarTruthTableCondition_16)
    |     aFcnTruthTableAction_3();
    | elseif (aVarTruthTableCondition_17)
    |     aFcnTruthTableAction_6();
    | elseif (aVarTruthTableCondition_18)
    |     aFcnTruthTableAction_3();
    | else % Default
    |     aFcnTruthTableAction_1();
    | end
    | 
    | function aFcnTruthTableAction_1()
    | 
    | % WeightShift
    | 
    | poseBML=encStr2Arr('<?xml version="1.0" ?><act><bml><animation name="ChrBrad@Idle01_WeightShift01" /></bml></act>');
    | 
    | function aFcnTruthTableAction_2()
    | 
    | % ScratchChest
    | 
    | poseBML=encStr2Arr('<?xml version="1.0" ?><act><bml><animation name="ChrRachel_ChrBrad@Idle01_ScratchChest01" /></bml></act>');
    | 
    | function aFcnTruthTableAction_3()
    | 
    | % ScratchHead
    | 
    | poseBML=encStr2Arr('<?xml version="1.0" ?><act><bml><animation name="ChrBrad@Idle01_ScratchHeadLf01" /></bml></act>');
    | 
    | function aFcnTruthTableAction_4()
    | 
    | % ShoulderStretchUpDown
    | 
    | poseBML=encStr2Arr('<?xml version="1.0" ?><act><bml><animation name="ChrBrad@Idle01_ShoulderStretch01" /></bml></act>');
    | 
    | function aFcnTruthTableAction_5()
    | 
    | % scratchtemple(head)
    | 
    | poseBML=encStr2Arr('<?xml version="1.0" ?><act><bml><animation name="ChrRachel_ChrBrad@Idle01_ScratchTempleLf01" /></bml></act>');
    | 
    | function aFcnTruthTableAction_6()
    | 
    | % SqueezeHand01
    | 
    | poseBML=encStr2Arr('<?xml version="1.0" ?><act><bml><animation name="ChrBrad@Idle01_SqueezeHand01" /></bml></act>');
    | 
    | function aFcnTruthTableAction_7()
    | 
    | % WeightShift2
    | 
    | poseBML=encStr2Arr('<?xml version="1.0" ?><act><bml><animation name="ChrBrad@Idle01_WeightShift02" /></bml></act>');
    | 
    | function aFcnTruthTableAction_8()
    | 
    | % Idle01_ToIdle02
    | 
    | poseBML=encStr2Arr('<?xml version="1.0" ?><act><bml><animation name="ChrBrad@Idle01_ToIdle02" /></bml></act>');
  function poseBML=initialPoseTable(bmlID):
    | function poseBML=initialPoseTable(bmlID)
    | 
    | aVarTruthTableCondition_1 = false;
    | aVarTruthTableCondition_2 = false;
    | aVarTruthTableCondition_3 = false;
    | 
    | 
    | 
    | aVarTruthTableCondition_1 = logical(bmlID==1);
    | 
    | 
    | aVarTruthTableCondition_2 = logical(bmlID==2);
    | 
    | 
    | aVarTruthTableCondition_3 = logical(bmlID==3);
    | 
    | if (aVarTruthTableCondition_1)
    |     aFcnTruthTableAction_1();
    | elseif (aVarTruthTableCondition_2)
    |     aFcnTruthTableAction_2();
    | elseif (aVarTruthTableCondition_3)
    |     aFcnTruthTableAction_1();
    | else % Default
    |     aFcnTruthTableAction_1();
    | end
    | 
    | function aFcnTruthTableAction_1()
    | 
    | % saccadeFinish
    | 
    | poseBML=encStr2Arr('<?xml version="1.0" ?><act><bml><saccade finish="true"/></bml></act>');
    | 
    | function aFcnTruthTableAction_2()
    | 
    | % neutralHeadGaze
    | 
    | poseBML=encStr2Arr('<?xml version="1.0" ?><act><bml><gaze target="camera" sbm:time-hint="0.2"/></bml></act>');
  function poseBML = successTable(bmlID):
    | function poseBML = successTable(bmlID)
    | 
    | aVarTruthTableCondition_1 = false;
    | aVarTruthTableCondition_2 = false;
    | aVarTruthTableCondition_3 = false;
    | 
    | 
    | % smile
    | 
    | aVarTruthTableCondition_1 = logical(bmlID==1);
    | 
    | % HeadChestUp
    | 
    | aVarTruthTableCondition_2 = logical(bmlID==2);
    | 
    | % browUp
    | 
    | aVarTruthTableCondition_3 = logical(bmlID==3);
    | 
    | if (aVarTruthTableCondition_1)
    |     aFcnTruthTableAction_1();
    | elseif (aVarTruthTableCondition_2)
    |     aFcnTruthTableAction_2();
    | elseif (aVarTruthTableCondition_3)
    |     aFcnTruthTableAction_3();
    | else % Default
    |     aFcnTruthTableAction_1();
    | end
    | 
    | function aFcnTruthTableAction_1()
    | 
    | % smile
    | 
    | poseBML=encStr2Arr('<?xml version="1.0" ?><act><bml><face amount="1" au="12" end="8" relax="6" side="BOTH" start="0" stroke="3" type="facs"/><face amount="0.5" au="6" end="8" relax="6" side="BOTH" start="0" stroke="3" type="facs"/></bml></act>');
    | 
    | function aFcnTruthTableAction_2()
    | 
    | % HeadChestUp
    | 
    | poseBML=encStr2Arr('<?xml version="1.0" ?><act><bml><gaze angle="12" direction="UP" sbm:joint-range="HEAD CHEST" sbm:time-hint="0.3" target="camera"/></bml></act>');
    | 
    | function aFcnTruthTableAction_3()
    | 
    | % browUp
    | 
    | poseBML=encStr2Arr('<?xml version="1.0" ?><act><bml><face amount="0.3" au="1" end="6" side="BOTH" start="0" type="facs"/><face amount="0.8"  au="2" end="6" side="BOTH" start="0" type="facs"/></bml></act>');

== stateflow chart lib_affectiveChar_scenario/pointToTarget ==
  state stateIdle
    entry: sendBML(cmdBML_idle());
  state stateCalculateUserStatus
  state sendBML(arg) [function]
  state statePointRight
    entry:
    sendBML(cmdBML_pointRt());
    agentState=1
  state statePointLeft
    entry:
    sendBML(cmdBML_pointLf());
    agentState=2
  state stateTarget
    entry:
    sendBML(cmdBML_target());
    agentState=3
  (default) -> stateIdle
  stateTarget -> stateIdle : after(2,secs)
  stateIdle -> stateCalculateUserStatus : after(1,secs)
  statePointLeft -> stateIdle : after(2,secs)
  statePointRight -> stateIdle : after(2,secs)
  stateCalculateUserStatus -> statePointRight [order 2] : after(1,secs)[xd<=0]
  stateCalculateUserStatus -> statePointLeft [order 1] : after(1,secs)[xd>0]
  stateCalculateUserStatus -> stateTarget [order 3] : after(1,secs)[xd==0]
  data: arg function_input double size=[256 1]; xd input double size=1; agentState output double size=1 =-1
  events: secs input RISING_EDGE_EVENT
